simulink model "test_sed"  (R2016b)
settings: Solver=VariableStepAuto  StartTime=0.0  StopTime=inf  RelTol=1e-3
settings Model: Creator=emiliendurif  LastModifiedBy=emiliendurif

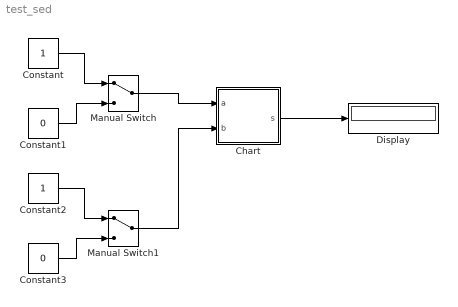
== system test_sed ==
  Chart : Stateflow chart  TreatAsAtomicUnit=on
  Constant : Constant
  Constant1 : Constant  Value=0
  Constant2 : Constant
  Constant3 : Constant  Value=0
  Display : Display
  Manual Switch : ManualSwitch
  Manual Switch1 : ManualSwitch
  wires:
  Constant/1 -> Manual Switch/1
  Constant1/1 -> Manual Switch/2
  Constant2/1 -> Manual Switch1/1
  Constant3/1 -> Manual Switch1/2
  Manual Switch/1 -> Chart/1(a)
  Manual Switch1/1 -> Chart/2(b)
  Chart/1(s) -> Display/1

== stateflow chart test_sed/Chart ==
  state e1
    en:s=0
  state e2
    en:s=1
  (default) -> e1
  e1 -> e2 : [a&b]
  e2 -> e1 : [!(a&b)]
  data: a input; b input; s output
